simulink model "gm_uz_inverter_3phgm"  (R2021b)
settings: Solver=FixedStepDiscrete  StartTime=0.0  StopTime=0.6  FixedStep=Auto  RelTol=1e-3
InitFcn:
  | load('C:\Users\valen\Documents\repos\UZ\ultrazohm_sw\ip_cores\uz_inverter_3ph\sschdl\uz_inverter_3ph\stateSpaceParameters.mat');
undefined symbols (not defined in the file or in its folder): g1, g2, g3, g4, g5, g6, i_a, i_b, i_c, pslcontrol, ts
libraries: hdlmdlgenlib x20, hdlssclib x2
settings Model: Creator=LENOVO  LastModifiedBy=valen
settings SolverCC: AlgebraicLoopSolver=TrustRegion
settings DataIOCC: LimitDataPoints=on  SaveOutput=off  SaveTime=off
settings OptimizationCC: BlockReduction=off  ConditionallyExecuteInputs=off  DefaultParameterBehavior=Inlined  InheritOutputTypeSmallerThanSingle=on  LifeSpan=inf
settings DebuggingCC: AlgebraicLoopMsg=error  InheritedTsInSrcMsg=none  SingleTaskRateTransMsg=error  AllowSymbolicDim=off  StrictBusMsg=ErrorOnBusTreatedAsVector  SFUnexpectedBacktrackingDiag=warning  SFNoUnconditionalDefaultTransitionDiag=warning  SFExecutionAtInitializationDiag=none  SFMachineParentedDataDiag=warning  ArithmeticOperatorsInVariantConditions=warning
settings HardwareCC: ProdBitPerPointer=32  ProdBitPerSizeT=32  ProdBitPerPtrDiffT=32  ProdLargestAtomicFloat=None  ProdIntDivRoundTo=Undefined  ProdEndianess=Unspecified  ProdWordSize=32  ProdHWDeviceType=ASIC/FPGA->ASIC/FPGA  ProdEqTarget=off
settings SFSimCC: SimUseLocalCustomCode=off  CustomCodeUndefinedFunction=UseInterfaceOnly
settings RTWCC: RTWUseLocalCustomCode=off
settings CodeAppCC: StateflowObjectComments=on
settings GRTTargetCC: TargetLangStandard=C89/C90 (ANSI)
settings ConfigComp: CovScope=ReferencedModels  CovMetricSettings=dw  CovSaveCumulativeToWorkspaceVar=on  CovSaveSingleToWorkspaceVar=on  CovExternalEMLEnable=off  CovSFcnEnable=off

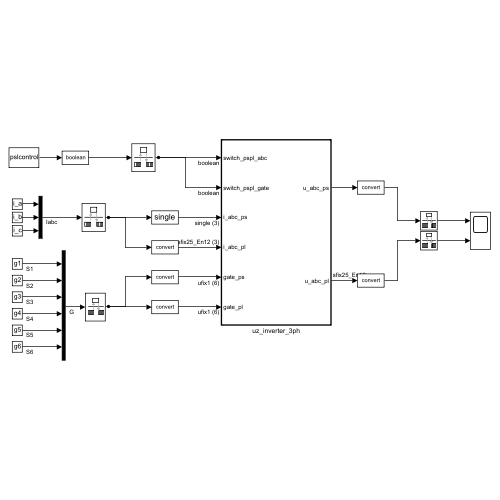
[thumbnail: Simulink's stored preview of the top-level diagram]
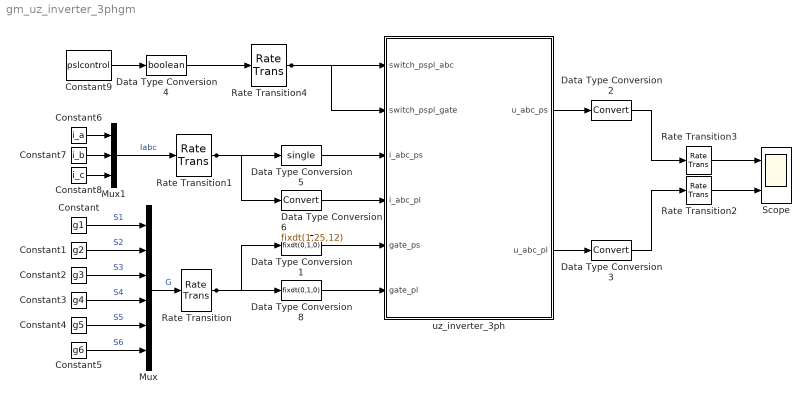
== system gm_uz_inverter_3phgm ==
  Constant : Constant  Value=g1  SampleTime=ts
  Constant1 : Constant  Value=g2  SampleTime=ts
  Constant2 : Constant  Value=g3  SampleTime=ts
  Constant3 : Constant  Value=g4  SampleTime=ts
  Constant4 : Constant  Value=g5  SampleTime=ts
  Constant5 : Constant  Value=g6  SampleTime=ts
  Constant6 : Constant  Value=i_a  SampleTime=ts
  Constant7 : Constant  Value=i_b  SampleTime=ts
  Constant8 : Constant  Value=i_c  SampleTime=ts
  Constant9 : Constant  Value=pslcontrol
  Data Type Conversion1 : DataTypeConversion  OutMin=0  OutMax=1  OutDataTypeStr=fixdt(0,1,0)  RndMeth=Nearest
  Data Type Conversion2 : DataTypeConversion
  Data Type Conversion3 : DataTypeConversion
  Data Type Conversion4 : DataTypeConversion  OutDataTypeStr=boolean
  Data Type Conversion5 : DataTypeConversion  OutDataTypeStr=single  RndMeth=Nearest
  Data Type Conversion6 : DataTypeConversion  OutDataTypeStr=fixdt(1,25,12)  RndMeth=Nearest
  Data Type Conversion8 : DataTypeConversion  OutMin=0  OutMax=1  OutDataTypeStr=fixdt(0,1,0)  RndMeth=Nearest
  Mux : Mux  Inputs=6
  Mux1 : Mux  Inputs=3
  Rate Transition{,1..4} (5 alike) : RateTransition  OutPortSampleTime=ts
  Scope : Scope  NumInputPorts=2
  uz_inverter_3ph : Subsystem  TreatAsAtomicUnit=on
  wires:
  Data Type Conversion5/1 -> uz_inverter_3ph/3(i_abc_ps)
  Data Type Conversion1/1 -> uz_inverter_3ph/5(gate_ps)
  Rate Transition/1 -> Data Type Conversion1/1, Data Type Conversion8/1
  Data Type Conversion8/1 -> uz_inverter_3ph/6(gate_pl)
  Data Type Conversion6/1 -> uz_inverter_3ph/4(i_abc_pl)
  Rate Transition1/1 -> Data Type Conversion6/1, Data Type Conversion5/1
  Constant/1 -> Mux/1  "S1"
  Constant7/1 -> Mux1/2
  Constant1/1 -> Mux/2  "S2"
  Constant6/1 -> Mux1/1
  Constant8/1 -> Mux1/3
  Mux/1 -> Rate Transition/1  "G"
  Mux1/1 -> Rate Transition1/1  "Iabc"
  Constant3/1 -> Mux/4  "S4"
  Constant5/1 -> Mux/6  "S6"
  Constant4/1 -> Mux/5  "S5"
  Constant2/1 -> Mux/3  "S3"
  Constant9/1 -> Data Type Conversion4/1
  Rate Transition4/1 -> uz_inverter_3ph/2(switch_pspl_gate), uz_inverter_3ph/1(switch_pspl_abc)
  Data Type Conversion4/1 -> Rate Transition4/1
  Rate Transition2/1 -> Scope/2
  Rate Transition3/1 -> Scope/1
  Data Type Conversion2/1 -> Rate Transition3/1
  Data Type Conversion3/1 -> Rate Transition2/1
  uz_inverter_3ph/2(u_abc_pl) -> Data Type Conversion3/1
  uz_inverter_3ph/1(u_abc_ps) -> Data Type Conversion2/1

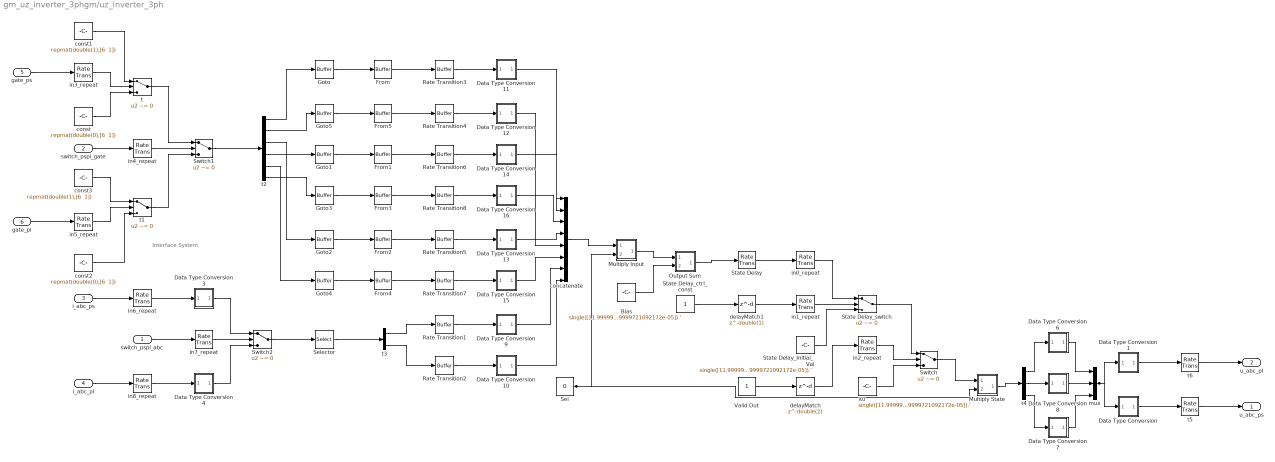
== system gm_uz_inverter_3phgm/uz_inverter_3ph ==
  note: Interface System
  switch_pspl_abc : Inport  OutDataTypeStr=boolean  PortDimensions=1  SampleTime=5e-07
  switch_pspl_gate : Inport  Port=2  OutDataTypeStr=boolean  PortDimensions=1  SampleTime=5e-07
  i_abc_ps : Inport  Port=3  OutDataTypeStr=single  PortDimensions=[3]  SampleTime=5e-07
  i_abc_pl : Inport  Port=4  OutDataTypeStr=fixdt(1, 25, 12)  PortDimensions=[3]  SampleTime=5e-07
  gate_ps : Inport  Port=5  OutDataTypeStr=fixdt(0, 1, 0)  PortDimensions=[6]  SampleTime=5e-07  LockScale=on
  gate_pl : Inport  Port=6  OutDataTypeStr=fixdt(0, 1, 0)  PortDimensions=[6]  SampleTime=5e-07
  Bias : Constant  Value=single([11.99999713897705 -11.99999713897705 0 -0.0002399999793851748 2.399999721092172e-05 -0.00012 1.2e-05 -2.6399995037285073e-11 0.00026399994385428727 0.00026399994385428727 1.2e-05 2.399999721092172e-05]).'  OutDataTypeStr=single  SampleTime=1e-08
  Data Type Conversion : Subsystem
      mask Display: disp('NFP\nconv');
  Data Type Conversion1 : Subsystem
      mask Display: disp('NFP\nconv');
  Data Type Conversion10 : Subsystem
      mask Display: disp('NFP\nconv');
  Data Type Conversion11 : Subsystem
      mask Display: disp('NFP\nconv');
  Data Type Conversion12 : Subsystem
      mask Display: disp('NFP\nconv');
  Data Type Conversion13 : Subsystem
      mask Display: disp('NFP\nconv');
  Data Type Conversion14 : Subsystem
      mask Display: disp('NFP\nconv');
  Data Type Conversion15 : Subsystem
      mask Display: disp('NFP\nconv');
  Data Type Conversion16 : Subsystem
      mask Display: disp('NFP\nconv');
  Data Type Conversion3 : Subsystem
      mask Display: disp('NFP\nconv');
  Data Type Conversion4 : Subsystem
      mask Display: disp('NFP\nconv');
  Data Type Conversion6 : Subsystem
      mask Display: disp('NFP\nconv');
  Data Type Conversion7 : Subsystem
      mask Display: disp('NFP\nconv');
  Data Type Conversion8 : Subsystem
      mask Display: disp('NFP\nconv');
  Data Type Conversion9 : Subsystem
      mask Display: disp('NFP\nconv');
  From{,1..5} (6 alike) : hdlmdlgenlib/Buffer
      settings: SourceProductBaseCode=SL
  Goto{,1..5} (6 alike) : hdlmdlgenlib/Buffer
      settings: SourceProductBaseCode=SL
  Multiply Input : Subsystem
      mask Display: disp('NFP\nSparseConstMultiply');
  Multiply State : Subsystem
      mask Display: disp('NFP\nSparseConstMultiply');
  Output Sum : Subsystem
      mask Display: disp('NFP\nadd');
  Rate Transition{1..8} (8 alike) : hdlmdlgenlib/Buffer
      settings: SourceProductBaseCode=SL
  Sel : Constant  Value=0  OutDataTypeStr=uint32  SampleTime=1e-08
  Selector : Selector  SampleTime=1e-08  IndexOptions=Index vector (dialog)  Indices=double([1 2])  OutputSizes=double(1)
  State Delay : RateTransition  OutPortSampleTimeOpt=Multiple of input port sample time  OutPortSampleTimeMultiple=50
  State Delay_Initial_Val : Constant  Value=single([11.99999713897705 -11.99999713897705 6.543061643369901e-16 -0.0002399999793851748 2.399999721092172e-05 -0.00012 1.2e-05 -2.6399995037285073e-11 0.00026399994385428727 0.00026399994385428727 1.2e-05 2.399999721092172e-05]).'  OutDataTypeStr=single  SampleTime=1e-08
  State Delay_ctrl_const : Constant  OutDataTypeStr=boolean  SampleTime=5e-07
  State Delay_switch : Switch  Criteria=u2 ~= 0  Threshold=double(0)  OutDataTypeStr=single  SampleTime=1e-08
  Switch : Switch  Criteria=u2 ~= 0  Threshold=double(0)  OutDataTypeStr=single  SampleTime=1e-08
  Switch1 : Switch  Criteria=u2 ~= 0  Threshold=double(0)  OutDataTypeStr=double  SampleTime=1e-08
  Switch2 : Switch  Criteria=u2 ~= 0  Threshold=double(0)  OutDataTypeStr=double  SampleTime=1e-08
  Valid Out : Constant  OutDataTypeStr=boolean  SampleTime=5e-07
  X0 : Constant  Value=single([11.99999713897705 -11.99999713897705 6.543061643369901e-16 -0.0002399999793851748 2.399999721092172e-05 -0.00012 1.2e-05 -2.6399995037285073e-11 0.00026399994385428727 0.00026399994385428727 1.2e-05 2.399999721092172e-05]).'  OutDataTypeStr=single  SampleTime=1e-08
  concatenate : Concatenate  NumInputs=8
  const : Constant  Value="repmat(double(0),[6  1])"  OutDataTypeStr=double  SampleTime=1e-08
  const1 : Constant  Value="repmat(double(1),[6  1])"  OutDataTypeStr=double  SampleTime=1e-08
  const2 : Constant  Value="repmat(double(0),[6  1])"  OutDataTypeStr=double  SampleTime=1e-08
  const3 : Constant  Value="repmat(double(1),[6  1])"  OutDataTypeStr=double  SampleTime=1e-08
  delayMatch : Delay  DelayLength=double(2)  InitialCondition=0  SampleTime=5e-07
  delayMatch1 : Delay  DelayLength=double(1)  InitialCondition=0  SampleTime=5e-07
  in0_repeat : RateTransition  Integrity=off  Deterministic=off  OutPortSampleTimeOpt=Multiple of input port sample time  OutPortSampleTimeMultiple=1/50
  in1_repeat : RateTransition  Integrity=off  Deterministic=off  OutPortSampleTimeOpt=Multiple of input port sample time  OutPortSampleTimeMultiple=1/50
  in2_repeat : RateTransition  Integrity=off  Deterministic=off  OutPortSampleTimeOpt=Multiple of input port sample time  OutPortSampleTimeMultiple=1/50
  in3_repeat : RateTransition  Integrity=off  Deterministic=off  OutPortSampleTimeOpt=Multiple of input port sample time  OutPortSampleTimeMultiple=1/50
  in4_repeat : RateTransition  Integrity=off  Deterministic=off  OutPortSampleTimeOpt=Multiple of input port sample time  OutPortSampleTimeMultiple=1/50
  in5_repeat : RateTransition  Integrity=off  Deterministic=off  OutPortSampleTimeOpt=Multiple of input port sample time  OutPortSampleTimeMultiple=1/50
  in6_repeat : RateTransition  Integrity=off  Deterministic=off  OutPortSampleTimeOpt=Multiple of input port sample time  OutPortSampleTimeMultiple=1/50
  in7_repeat : RateTransition  Integrity=off  Deterministic=off  OutPortSampleTimeOpt=Multiple of input port sample time  OutPortSampleTimeMultiple=1/50
  in8_repeat : RateTransition  Integrity=off  Deterministic=off  OutPortSampleTimeOpt=Multiple of input port sample time  OutPortSampleTimeMultiple=1/50
  mux : Mux  Inputs=3
  t : Switch  Criteria=u2 ~= 0  Threshold=double(0)  OutDataTypeStr=double  SampleTime=1e-08
  t1 : Switch  Criteria=u2 ~= 0  Threshold=double(0)  OutDataTypeStr=double  SampleTime=1e-08
  t2 : Demux  Outputs=6
  t3 : Demux  Outputs=2
  t4 : Demux  Outputs=3
  t5 : RateTransition  OutPortSampleTimeOpt=Multiple of input port sample time  OutPortSampleTimeMultiple=50
  t6 : RateTransition  OutPortSampleTimeOpt=Multiple of input port sample time  OutPortSampleTimeMultiple=50
  u_abc_ps : Outport  SampleTime=5e-07
  u_abc_pl : Outport  Port=2  OutDataTypeStr=fixdt(1,25,12)  SampleTime=5e-07
  wires:
  switch_pspl_abc/1 -> in7_repeat/1
  switch_pspl_gate/1 -> in4_repeat/1
  i_abc_ps/1 -> in6_repeat/1
  i_abc_pl/1 -> in8_repeat/1
  gate_ps/1 -> in3_repeat/1
  gate_pl/1 -> in5_repeat/1
  delayMatch/1 -> in2_repeat/1
  delayMatch1/1 -> in1_repeat/1
  t5/1 -> u_abc_ps/1
  t6/1 -> u_abc_pl/1
  State Delay/1 -> in0_repeat/1
  Valid Out/1 -> delayMatch/1
  State Delay_ctrl_const/1 -> delayMatch1/1
  in0_repeat/1 -> State Delay_switch/1
  in1_repeat/1 -> State Delay_switch/2
  in2_repeat/1 -> Switch/2
  in3_repeat/1 -> t/2
  in4_repeat/1 -> Switch1/2
  in5_repeat/1 -> t1/2
  in6_repeat/1 -> Data Type Conversion3/1(In1)
  in7_repeat/1 -> Switch2/2
  in8_repeat/1 -> Data Type Conversion4/1(In1)
  State Delay_Initial_Val/1 -> State Delay_switch/3
  State Delay_switch/1 -> Switch/1
  X0/1 -> Switch/3
  Switch/1 -> Multiply State/1(In1)
  Bias/1 -> Output Sum/2(In2)
  Rate Transition4/1 -> Data Type Conversion12/1(In1)
  From5/1 -> Rate Transition4/1
  Goto5/1 -> From5/1
  Rate Transition5/1 -> Data Type Conversion13/1(In1)
  From2/1 -> Rate Transition5/1
  Goto2/1 -> From2/1
  Rate Transition6/1 -> Data Type Conversion14/1(In1)
  From1/1 -> Rate Transition6/1
  Goto1/1 -> From1/1
  Rate Transition7/1 -> Data Type Conversion15/1(In1)
  From4/1 -> Rate Transition7/1
  Goto4/1 -> From4/1
  Rate Transition8/1 -> Data Type Conversion16/1(In1)
  From3/1 -> Rate Transition8/1
  Goto3/1 -> From3/1
  t/1 -> Switch1/1
  t1/1 -> Switch1/3
  Switch1/1 -> t2/1
  Goto/1 -> From/1
  From/1 -> Rate Transition3/1
  Rate Transition3/1 -> Data Type Conversion11/1(In1)
  Rate Transition2/1 -> Data Type Conversion10/1(In1)
  Switch2/1 -> Selector/1
  Selector/1 -> t3/1
  Rate Transition1/1 -> Data Type Conversion9/1(In1)
  concatenate/1 -> Multiply Input/1(In1)
  Sel/1 -> Multiply State/2(In2), Multiply Input/2(In2)
  mux/1 -> Data Type Conversion/1(In1), Data Type Conversion1/1(In1)
  const/1 -> t/3
  const1/1 -> t/1
  const2/1 -> t1/3
  const3/1 -> t1/1
  t2/1 -> Goto/1
  t2/2 -> Goto5/1
  t2/3 -> Goto2/1
  t2/4 -> Goto1/1
  t2/5 -> Goto4/1
  t2/6 -> Goto3/1
  t3/1 -> Rate Transition1/1
  t3/2 -> Rate Transition2/1
  t4/1 -> Data Type Conversion6/1(In1)
  t4/2 -> Data Type Conversion8/1(In1)
  t4/3 -> Data Type Conversion7/1(In1)
  Data Type Conversion1/1(Out1) -> t6/1
  Data Type Conversion8/1(Out1) -> mux/2
  Data Type Conversion7/1(Out1) -> mux/3
  Output Sum/1(Out1) -> State Delay/1
  Data Type Conversion12/1(Out1) -> concatenate/5
  Data Type Conversion13/1(Out1) -> concatenate/4
  Data Type Conversion14/1(Out1) -> concatenate/2
  Data Type Conversion15/1(Out1) -> concatenate/6
  Data Type Conversion16/1(Out1) -> concatenate/3
  Data Type Conversion11/1(Out1) -> concatenate/1
  Data Type Conversion10/1(Out1) -> concatenate/8
  Data Type Conversion3/1(Out1) -> Switch2/1
  Data Type Conversion4/1(Out1) -> Switch2/3
  Data Type Conversion9/1(Out1) -> concatenate/7
  Multiply Input/1(Out1) -> Output Sum/1(In1)
  Multiply State/1(Out1) -> t4/1
  Data Type Conversion6/1(Out1) -> mux/1
  Data Type Conversion/1(Out1) -> t5/1

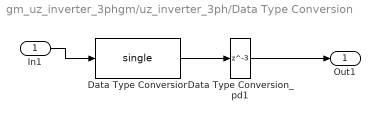
== system gm_uz_inverter_3phgm/uz_inverter_3ph/Data Type Conversion ==
  In1 : Inport
  Data Type Conversion : DataTypeConversion  OutDataTypeStr=single  RndMeth=Nearest  SampleTime=1e-08
  Data Type Conversion_pd1 : Delay  DelayLength=3
  Out1 : Outport
  wires:
  In1/1 -> Data Type Conversion/1
  Data Type Conversion/1 -> Data Type Conversion_pd1/1
  Data Type Conversion_pd1/1 -> Out1/1

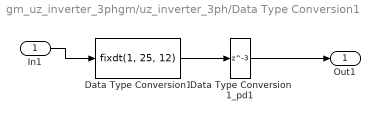
== system gm_uz_inverter_3phgm/uz_inverter_3ph/Data Type Conversion1 ==
  In1 : Inport
  Data Type Conversion1 : DataTypeConversion  OutDataTypeStr=fixdt(1, 25, 12)  RndMeth=Nearest  SampleTime=1e-08
  Data Type Conversion1_pd1 : Delay  DelayLength=3
  Out1 : Outport
  wires:
  In1/1 -> Data Type Conversion1/1
  Data Type Conversion1/1 -> Data Type Conversion1_pd1/1
  Data Type Conversion1_pd1/1 -> Out1/1

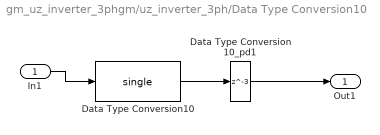
== system gm_uz_inverter_3phgm/uz_inverter_3ph/Data Type Conversion10 ==
  In1 : Inport
  Data Type Conversion10 : DataTypeConversion  OutDataTypeStr=single  RndMeth=Nearest  SampleTime=1e-08
  Data Type Conversion10_pd1 : Delay  DelayLength=3
  Out1 : Outport
  wires:
  In1/1 -> Data Type Conversion10/1
  Data Type Conversion10/1 -> Data Type Conversion10_pd1/1
  Data Type Conversion10_pd1/1 -> Out1/1

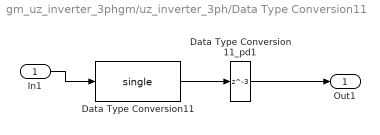
== system gm_uz_inverter_3phgm/uz_inverter_3ph/Data Type Conversion11 ==
  In1 : Inport
  Data Type Conversion11 : DataTypeConversion  OutDataTypeStr=single  RndMeth=Nearest  SampleTime=1e-08
  Data Type Conversion11_pd1 : Delay  DelayLength=3
  Out1 : Outport
  wires:
  In1/1 -> Data Type Conversion11/1
  Data Type Conversion11/1 -> Data Type Conversion11_pd1/1
  Data Type Conversion11_pd1/1 -> Out1/1

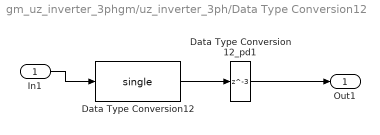
== system gm_uz_inverter_3phgm/uz_inverter_3ph/Data Type Conversion12 ==
  In1 : Inport
  Data Type Conversion12 : DataTypeConversion  OutDataTypeStr=single  RndMeth=Nearest  SampleTime=1e-08
  Data Type Conversion12_pd1 : Delay  DelayLength=3
  Out1 : Outport
  wires:
  In1/1 -> Data Type Conversion12/1
  Data Type Conversion12/1 -> Data Type Conversion12_pd1/1
  Data Type Conversion12_pd1/1 -> Out1/1

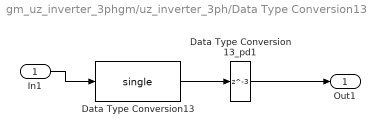
== system gm_uz_inverter_3phgm/uz_inverter_3ph/Data Type Conversion13 ==
  In1 : Inport
  Data Type Conversion13 : DataTypeConversion  OutDataTypeStr=single  RndMeth=Nearest  SampleTime=1e-08
  Data Type Conversion13_pd1 : Delay  DelayLength=3
  Out1 : Outport
  wires:
  In1/1 -> Data Type Conversion13/1
  Data Type Conversion13/1 -> Data Type Conversion13_pd1/1
  Data Type Conversion13_pd1/1 -> Out1/1

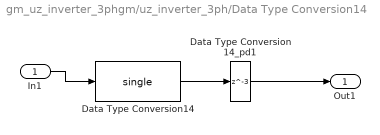
== system gm_uz_inverter_3phgm/uz_inverter_3ph/Data Type Conversion14 ==
  In1 : Inport
  Data Type Conversion14 : DataTypeConversion  OutDataTypeStr=single  RndMeth=Nearest  SampleTime=1e-08
  Data Type Conversion14_pd1 : Delay  DelayLength=3
  Out1 : Outport
  wires:
  In1/1 -> Data Type Conversion14/1
  Data Type Conversion14/1 -> Data Type Conversion14_pd1/1
  Data Type Conversion14_pd1/1 -> Out1/1

== system gm_uz_inverter_3phgm/uz_inverter_3ph/Data Type Conversion15 ==
  In1 : Inport
  Data Type Conversion15 : DataTypeConversion  OutDataTypeStr=single  RndMeth=Nearest  SampleTime=1e-08
  Data Type Conversion15_pd1 : Delay  DelayLength=3
  Out1 : Outport
  wires:
  In1/1 -> Data Type Conversion15/1
  Data Type Conversion15/1 -> Data Type Conversion15_pd1/1
  Data Type Conversion15_pd1/1 -> Out1/1

== system gm_uz_inverter_3phgm/uz_inverter_3ph/Data Type Conversion16 ==
  In1 : Inport
  Data Type Conversion16 : DataTypeConversion  OutDataTypeStr=single  RndMeth=Nearest  SampleTime=1e-08
  Data Type Conversion16_pd1 : Delay  DelayLength=3
  Out1 : Outport
  wires:
  In1/1 -> Data Type Conversion16/1
  Data Type Conversion16/1 -> Data Type Conversion16_pd1/1
  Data Type Conversion16_pd1/1 -> Out1/1

== system gm_uz_inverter_3phgm/uz_inverter_3ph/Data Type Conversion3 ==
  In1 : Inport
  Data Type Conversion3 : DataTypeConversion  OutDataTypeStr=double  RndMeth=Nearest  SampleTime=1e-08
  Data Type Conversion3_pd1 : Delay  DelayLength=3
  Out1 : Outport
  wires:
  In1/1 -> Data Type Conversion3/1
  Data Type Conversion3/1 -> Data Type Conversion3_pd1/1
  Data Type Conversion3_pd1/1 -> Out1/1

== system gm_uz_inverter_3phgm/uz_inverter_3ph/Data Type Conversion4 ==
  In1 : Inport
  Data Type Conversion4 : DataTypeConversion  OutDataTypeStr=double  RndMeth=Nearest  SampleTime=1e-08
  Data Type Conversion4_pd1 : Delay  DelayLength=3
  Out1 : Outport
  wires:
  In1/1 -> Data Type Conversion4/1
  Data Type Conversion4/1 -> Data Type Conversion4_pd1/1
  Data Type Conversion4_pd1/1 -> Out1/1

== system gm_uz_inverter_3phgm/uz_inverter_3ph/Data Type Conversion6 ==
  In1 : Inport
  Data Type Conversion6 : DataTypeConversion  OutDataTypeStr=double  RndMeth=Nearest  SampleTime=1e-08
  Data Type Conversion6_pd1 : Delay  DelayLength=3
  Out1 : Outport
  wires:
  In1/1 -> Data Type Conversion6/1
  Data Type Conversion6/1 -> Data Type Conversion6_pd1/1
  Data Type Conversion6_pd1/1 -> Out1/1

== system gm_uz_inverter_3phgm/uz_inverter_3ph/Data Type Conversion7 ==
  In1 : Inport
  Data Type Conversion7 : DataTypeConversion  OutDataTypeStr=double  RndMeth=Nearest  SampleTime=1e-08
  Data Type Conversion7_pd1 : Delay  DelayLength=3
  Out1 : Outport
  wires:
  In1/1 -> Data Type Conversion7/1
  Data Type Conversion7/1 -> Data Type Conversion7_pd1/1
  Data Type Conversion7_pd1/1 -> Out1/1

== system gm_uz_inverter_3phgm/uz_inverter_3ph/Data Type Conversion8 ==
  In1 : Inport
  Data Type Conversion8 : DataTypeConversion  OutDataTypeStr=double  RndMeth=Nearest  SampleTime=1e-08
  Data Type Conversion8_pd1 : Delay  DelayLength=3
  Out1 : Outport
  wires:
  In1/1 -> Data Type Conversion8/1
  Data Type Conversion8/1 -> Data Type Conversion8_pd1/1
  Data Type Conversion8_pd1/1 -> Out1/1

== system gm_uz_inverter_3phgm/uz_inverter_3ph/Data Type Conversion9 ==
  In1 : Inport
  Data Type Conversion9 : DataTypeConversion  OutDataTypeStr=single  RndMeth=Nearest  SampleTime=1e-08
  Data Type Conversion9_pd1 : Delay  DelayLength=3
  Out1 : Outport
  wires:
  In1/1 -> Data Type Conversion9/1
  Data Type Conversion9/1 -> Data Type Conversion9_pd1/1
  Data Type Conversion9_pd1/1 -> Out1/1

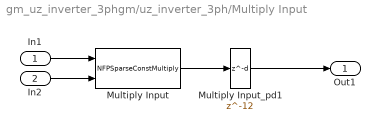
== system gm_uz_inverter_3phgm/uz_inverter_3ph/Multiply Input ==
  In1 : Inport
  In2 : Inport  Port=2
  Multiply Input : hdlssclib/NFPSparseConstMultiply  constMatrix="reshape(single([0 0 0 0 0 0 0 0 0 0 0 0 0 0 0 0 0 0 0 0 0 0 0 0 0 0 0 0 0 0 0 0 0 0 0 0 0 0 0 0 0 0 0 0 0 0 0 0 0 0 0 0 0 0 0 0 0 0 0 0 0 0 0 0 0 0 0 0 0 0 0 0 -0.009999997913837433 0 45454.5469 9.999997985232767e-08 -9.999998162868451e-09 0.4545454680919647 -0.04545454680919647 0 0 0.9999997615814209 0.04545454680919647 0 0 -0.009999997913837433 45454.5469 0 0 0.4545454680919647 -0.04545454680919647 9.999997985232767e-08 -0.9999997615814209 0 0.04545454680919647 9.999998162868451e-09]).', [12   8])"
      settings: SourceProductBaseCode=SL
  Multiply Input_pd1 : Delay  DelayLength=12
  Out1 : Outport
  wires:
  In1/1 -> Multiply Input/1
  In2/1 -> Multiply Input/2
  Multiply Input/1 -> Multiply Input_pd1/1
  Multiply Input_pd1/1 -> Out1/1

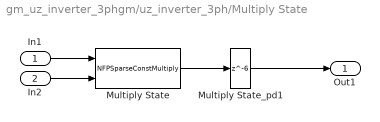
== system gm_uz_inverter_3phgm/uz_inverter_3ph/Multiply State ==
  In1 : Inport
  In2 : Inport  Port=2
  Multiply State : hdlssclib/NFPSparseConstMultiply  constMatrix="reshape(single([1 0 -1 0 1 0 0 0 0 0 0 0 0 0 0 0 0 0 0 0 0 0 0 0 0 0 0 0 0 0 0 0 0 0 0 0]).', [3  12])"
      settings: SourceProductBaseCode=SL
  Multiply State_pd1 : Delay  DelayLength=6
  Out1 : Outport
  wires:
  In1/1 -> Multiply State/1
  In2/1 -> Multiply State/2
  Multiply State/1 -> Multiply State_pd1/1
  Multiply State_pd1/1 -> Out1/1

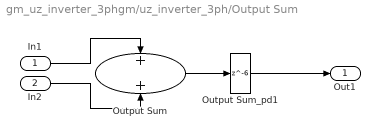
== system gm_uz_inverter_3phgm/uz_inverter_3ph/Output Sum ==
  In1 : Inport
  In2 : Inport  Port=2
  Output Sum : Sum  OutDataTypeStr=single  SampleTime=1e-08
  Output Sum_pd1 : Delay  DelayLength=6
  Out1 : Outport
  wires:
  In1/1 -> Output Sum/1
  In2/1 -> Output Sum/2
  Output Sum/1 -> Output Sum_pd1/1
  Output Sum_pd1/1 -> Out1/1
